simulink model "lab_part2"  (R2022a)
settings: Solver=ode45  StartTime=0.0  StopTime=3  MaxStep=0.001  RelTol=1e-3
values from neighbouring files (symbols this model uses):
  a = 2.5    [part3_plot.m]
  zeta = .6    (= 0.6)    [init.m]    (also in part3_plot.m)
settings Model: Creator=zhong  LastModifiedBy=zhong
settings DataIOCC: ExternalInput=a  InspectSignalLogs=on  ReturnWorkspaceOutputs=off

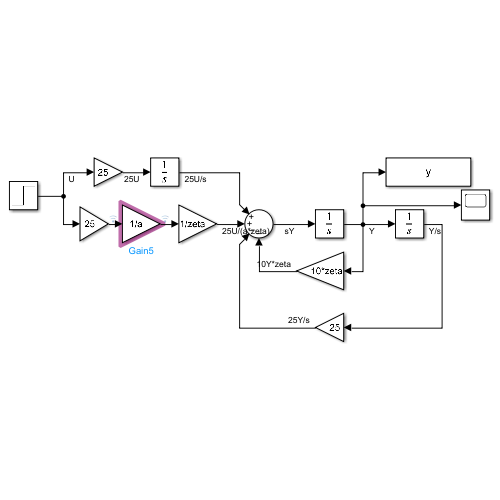
[thumbnail: Simulink's stored preview of the top-level diagram]
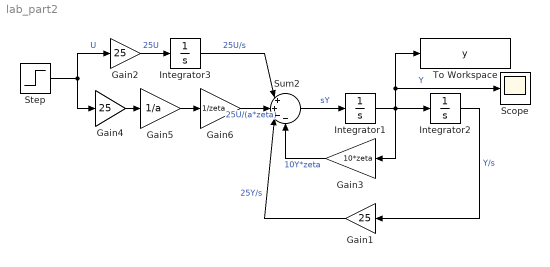
== system lab_part2 ==
  Gain1 : Gain  Gain=25
  Gain2 : Gain  Gain=25
  Gain3 : Gain  Gain=10*zeta
  Gain4 : Gain  Gain=25
  Gain5 : Gain  Gain=1/a
  Gain6 : Gain  Gain=1/zeta
  Integrator1 : Integrator
  Integrator2 : Integrator
  Integrator3 : Integrator
  Scope : Scope
  Step : Step  Time=0  SampleTime=0
  Sum2 : Sum  Inputs=|++--
  To Workspace : ToWorkspace  VariableName=y  SampleTime=-1
  wires:
  Integrator1/1 -> Gain3/1, Scope/1, To Workspace/1, Integrator2/1  "Y"
  Step/1 -> Gain2/1, Gain4/1  "U"
  Gain2/1 -> Integrator3/1  "25U"
  Sum2/1 -> Integrator1/1  "sY"
  Integrator2/1 -> Gain1/1  "Y/s"
  Integrator3/1 -> Sum2/1  "25U/s"
  Gain3/1 -> Sum2/4  "10Y*zeta"
  Gain1/1 -> Sum2/3  "25Y/s"
  Gain5/1 -> Gain6/1
  Gain6/1 -> Sum2/2  "25U/(a*zeta)"
  Gain4/1 -> Gain5/1
